simulink subsystem "Injector"  (R2020b)
settings: Solver=VariableStepAuto  StartTime=0.0  StopTime=10.0  RelTol=1e-3
model mask{dischargeCoeff=0.64}
  mask prompts: dischargeCoeff "Cd"
libraries: fl_lib x13, nesl_utility x3
settings Model: Creator=Edward  LastModifiedBy=Edward

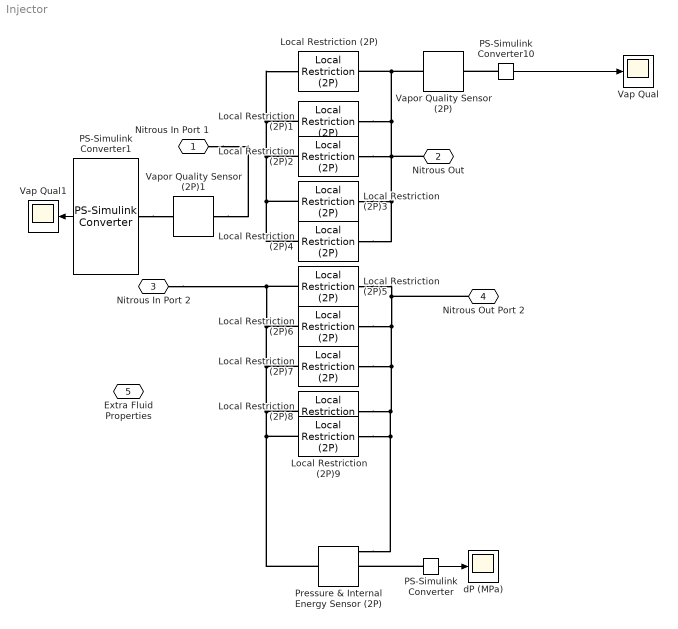
== system Injector ==
  Local Restriction (2P){,1..9} (10 alike) : fl_lib/Two-Phase Fluid/Elements/Local Restriction (2P)  restriction_area=Sim.injector.singleHoleA m^2  area=Sim.preInjectorPipe.crossSection m^2  Cd=dischargeCoeff  B_lam=0.999
      settings: SourceProductBaseCode=SS  InternalSimscapePortConfiguration="{\"Bottom\":[],\"Left\":[{\"id\":\"A\",\"label\":\"A\",\"type\":\"foundation.two_phase_fluid.two_phase_fluid\"}],\"Right\":[{\"id\":\"B\",\"label\":\"B\",\"type\":\"foundation.two_phase_fluid.two_phase_fluid\"}],\"Top\":[]}"
  PS-Simulink Converter : nesl_utility/PS-Simulink Converter  PhysicalDomain=network_engine_domain  SubClassName=ps_output  LeftPortType=input  RightPortType=output  PseudoPeriodic=off  Frequencies=[]  Unit=inherit  AffineConversion=off
  PS-Simulink Converter1 : nesl_utility/PS-Simulink Converter  PhysicalDomain=network_engine_domain  SubClassName=ps_output  LeftPortType=input  RightPortType=output  PseudoPeriodic=off  Frequencies=[]  Unit=inherit  AffineConversion=off
  PS-Simulink Converter10 : nesl_utility/PS-Simulink Converter  PhysicalDomain=network_engine_domain  SubClassName=ps_output  LeftPortType=input  RightPortType=output  PseudoPeriodic=off  Frequencies=[]  Unit=inherit  AffineConversion=off
  Pressure & Internal Energy Sensor (2P) : fl_lib/Two-Phase Fluid/Sensors/Pressure & Internal Energy Sensor (2P)
      settings: SourceProductBaseCode=SS  InternalSimscapePortConfiguration="{\"Bottom\":[],\"Left\":[{\"id\":\"A\",\"label\":\"A\",\"type\":\"foundation.two_phase_fluid.two_phase_fluid\"}],\"Right\":[{\"id\":\"B\",\"label\":\"B\",\"type\":\"foundation.two_phase_fluid.two_phase_fluid\"},{\"id\":\"P\",\"label\":\"P\",\"type\":\"output\"},{\"id\":\"U\",\"label\":\"U\",\"type\":\"output\"}],\"Top\":[]}"
  Vap Qual : Scope
  Vap Qual1 : Scope
  Vapor Quality Sensor (2P) : fl_lib/Two-Phase Fluid/Sensors/Vapor Quality Sensor (2P)  vapor_fraction_spec=foundation.enum.vapor_fraction_spec.quality
      settings: SourceProductBaseCode=SS  InternalSimscapePortConfiguration="{\"Bottom\":[],\"Left\":[{\"id\":\"A\",\"label\":\"A\",\"type\":\"foundation.two_phase_fluid.two_phase_fluid\"}],\"Right\":[{\"id\":\"X\",\"label\":\"X\",\"type\":\"output\"}],\"Top\":[]}"
  Vapor Quality Sensor (2P)1 : fl_lib/Two-Phase Fluid/Sensors/Vapor Quality Sensor (2P)  vapor_fraction_spec=foundation.enum.vapor_fraction_spec.quality
      settings: SourceProductBaseCode=SS  InternalSimscapePortConfiguration="{\"Bottom\":[],\"Left\":[{\"id\":\"A\",\"label\":\"A\",\"type\":\"foundation.two_phase_fluid.two_phase_fluid\"}],\"Right\":[{\"id\":\"X\",\"label\":\"X\",\"type\":\"output\"}],\"Top\":[]}"
  dP (MPa) : Scope
  Nitrous In Port 1 : PMIOPort  Side=Left
  Nitrous Out : PMIOPort  Port=2  Side=Right
  Nitrous In Port 2 : PMIOPort  Port=3  Side=Left
  Nitrous Out Port 2 : PMIOPort  Port=4  Side=Right
  Extra Fluid Properties : PMIOPort  Port=5  Side=Left
  wires:
  PS-Simulink Converter1/1 -> Vap Qual1/1
  PS-Simulink Converter10/1 -> Vap Qual/1
  PS-Simulink Converter/1 -> dP (MPa)/1
  connections:
  Local Restriction (2P)6/RConn1 -- Pressure & Internal Energy Sensor (2P)/RConn1 -- Local Restriction (2P)9/RConn1 -- Local Restriction (2P)8/RConn1 -- Local Restriction (2P)7/RConn1 -- Local Restriction (2P)5/RConn1 -- Nitrous Out Port 2/RConn1
  Local Restriction (2P)6/LConn1 -- Pressure & Internal Energy Sensor (2P)/LConn1 -- Local Restriction (2P)9/LConn1 -- Local Restriction (2P)8/LConn1 -- Local Restriction (2P)7/LConn1 -- Local Restriction (2P)5/LConn1 -- Nitrous In Port 2/RConn1
  Vapor Quality Sensor (2P)1/LConn1 -- Local Restriction (2P)4/LConn1 -- Local Restriction (2P)3/LConn1 -- Local Restriction (2P)2/LConn1 -- Local Restriction (2P)1/LConn1 -- Local Restriction (2P)/LConn1 -- Nitrous In Port 1/RConn1
  Local Restriction (2P)2/RConn1 -- Nitrous Out/RConn1 -- Local Restriction (2P)1/RConn1 -- Vapor Quality Sensor (2P)/LConn1 -- Local Restriction (2P)/RConn1 -- Local Restriction (2P)3/RConn1 -- Local Restriction (2P)4/RConn1
  PS-Simulink Converter1/LConn1 -- Vapor Quality Sensor (2P)1/RConn1
  PS-Simulink Converter10/LConn1 -- Vapor Quality Sensor (2P)/RConn1
  PS-Simulink Converter/LConn1 -- Pressure & Internal Energy Sensor (2P)/RConn2
